simulink model "test_increase_button_general"  (R2022b)
settings: Solver=FixedStepAuto  StartTime=0.0  StopTime=240  FixedStep=0.1  RelTol=1e-3
settings Model: Creator=alewi  LastModifiedBy=cristian
settings ConfigComp: CovEnable=on  RecordCoverage=on  CovModelRefEnable=on

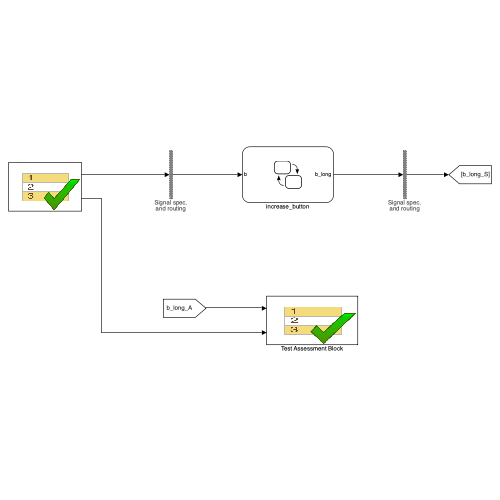
[thumbnail: Simulink's stored preview of the top-level diagram]
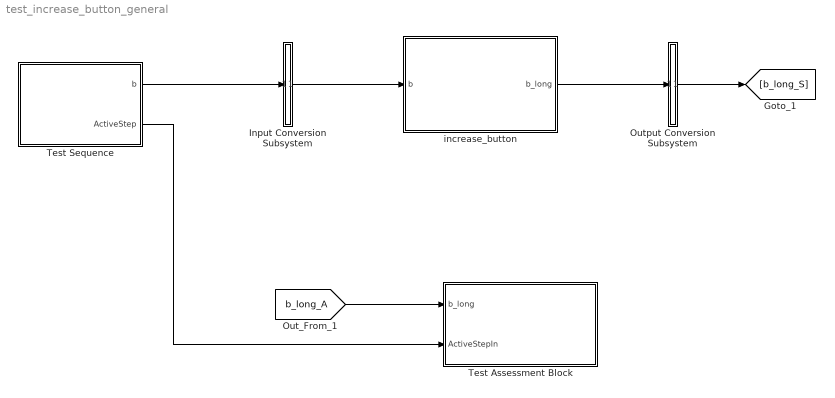
== system test_increase_button_general ==
  Input Conversion Subsystem : Subsystem  Tag=__SLT_ICS__  Description=|
      | Signal spec.
      | and routing
      settings: AttributesFormatString=%<Description>
  Output Conversion Subsystem : Subsystem  Tag=__SLT_OCS__  Description=|
      | Signal spec.
      | and routing
      settings: AttributesFormatString=%<Description>
  Test Assessment Block : Test Sequence  Tag=__SLT_ASMT__  TreatAsAtomicUnit=on
  Test Sequence : Test Sequence  TreatAsAtomicUnit=on
  increase_button : Stateflow chart  TreatAsAtomicUnit=on
  wires:
  Test Sequence/1(b) -> Input Conversion Subsystem/1(Inport_1)
  Output Conversion Subsystem/1(Outport_1) -> [b_long_S]
  Input Conversion Subsystem/1(Outport_1) -> increase_button/1(b)
  increase_button/1(b_long) -> Output Conversion Subsystem/1(Inport_1)
  Test Sequence/2(ActiveStep) -> Test Assessment Block/2(ActiveStepIn)
  [b_long_A] -> Test Assessment Block/1(b_long)

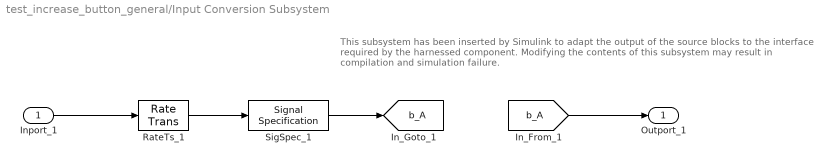
== system test_increase_button_general/Input Conversion Subsystem ==
  note: This subsystem has been inserted by Simulink to adapt the output of the source blocks to the interface required by the harnessed component.
      |  Modifying the contents of this subsystem may result in compilation and simulation failure.
  Inport_1 : Inport
  RateTs_1 : RateTransition  OutPortSampleTime=[-1, 0]
  SigSpec_1 : SignalSpecification  OutDataTypeStr=boolean  Dimensions=[1]  SampleTime=[-1, 0]
  Outport_1 : Outport
  tag scope: b_A=global
  wires:
  [b_A] -> Outport_1/1
  SigSpec_1/1 -> [b_A]
  RateTs_1/1 -> SigSpec_1/1
  Inport_1/1 -> RateTs_1/1

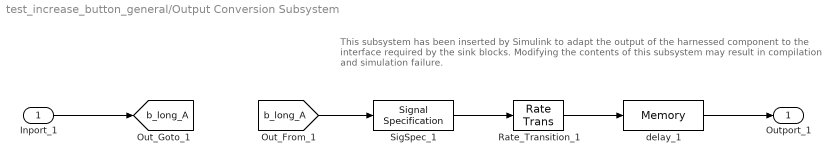
== system test_increase_button_general/Output Conversion Subsystem ==
  note: This subsystem has been inserted by Simulink to adapt the output of the harnessed component to the interface required by the sink blocks.
      |  Modifying the contents of this subsystem may result in compilation and simulation failure.
  Inport_1 : Inport
  Rate_Transition_1 : RateTransition  OutPortSampleTimeOpt=Inherit
  SigSpec_1 : SignalSpecification  OutDataTypeStr=boolean  Dimensions=[1]
  delay_1 : Memory
  Outport_1 : Outport
  tag scope: b_long_A=global
  wires:
  Inport_1/1 -> [b_long_A]
  [b_long_A] -> SigSpec_1/1
  SigSpec_1/1 -> Rate_Transition_1/1
  Rate_Transition_1/1 -> delay_1/1
  delay_1/1 -> Outport_1/1

== stateflow chart test_increase_button_general/Test Assessment Block ==
  state General
    state Run
      settings: description=Esecuzione test
      state Verify_G_Init
        verify(b_long == 1);
        settings: description=Inizialmente il bottone è rilasciato, per cui non è stato rilevato alcun long press.
      state Verify_G_ButtonPressed1
        settings: description=Bottone premuto
        state Verify_G_ButtonPressed1_1
          verify(b_long == 1);
          settings: description=Fino a che non passa 1 secondo, non viene rilevato alcun cambiamento nella potenza.
        state Verify_G_ButtonPressed1_2
          verify(b_long == 0);
          settings: description=Viene rilevata la pressione lunga.
        (default) -> Verify_G_ButtonPressed1_1
        Verify_G_ButtonPressed1_1 -> Verify_G_ButtonPressed1_2 : [
            | after(1,sec)
            | ]
      state Verify_G_ButtonReleased
        verify(b_long == 1);
        settings: description=La pressione lunga viene resettata.
      state Verify_G_ButtonPressed2
        settings: description=Bottone premuto
        state Verify_G_ButtonPressed2_1
          verify(b_long == 1)
          settings: description=Fino a che non passa 1 secondo, non viene rilevato alcun cambiamento nella potenza.
        state Verify_G_ButtonPressed2_2
          verify(b_long == 0);
          settings: description=Viene rilevata la pressione lunga.
        state Verify_G_ButtonPressed2_3
          verify(b_long == 1)
          settings: description=La pressione lunga viene resettata.
        (default) -> Verify_G_ButtonPressed2_1
        Verify_G_ButtonPressed2_1 -> Verify_G_ButtonPressed2_2 : [
            | after(1,sec)
            | ]
        Verify_G_ButtonPressed2_2 -> Verify_G_ButtonPressed2_3 : [
            | after(sampleTime,sec)
            | ]
      state Verify_G_ButtonReleased2
        verify(b_long == 1)
        settings: description=Il bottone è rilasciato, per cui non viene rilevato alcun long press
      state step_1_2
      (default) -> (junction 311)
      Run -> (junction 311)
      (junction 311) -> (junction 312) [order 1] : [ActiveStepIn == ActiveStepEnumH1.G_Init
          | ]
      (junction 312) -> Verify_G_Init [order 1] : [~in(General.Run.Verify_G_Init)]
      (junction 311) -> (junction 320) [order 2]
      (junction 312) -> (junction 315) [order 2]
      (junction 320) -> (junction 321) [order 1] : [ActiveStepIn == ActiveStepEnumH1.G_ButtonPressed
          | ]
      (junction 321) -> Verify_G_ButtonPressed1 [order 1] : [~in(General.Run.Verify_G_ButtonPressed1)]
      (junction 320) -> (junction 335) [order 2]
      (junction 321) -> (junction 324) [order 2]
      (junction 335) -> (junction 336) [order 1] : [ActiveStepIn == ActiveStepEnumH1.G_ButtonReleased
          | ]
      (junction 336) -> Verify_G_ButtonReleased [order 1] : [~in(General.Run.Verify_G_ButtonReleased)]
      (junction 335) -> (junction 343) [order 2]
      (junction 336) -> (junction 339) [order 2]
      (junction 343) -> (junction 344) [order 1] : [ActiveStepIn == ActiveStepEnumH1.G_ButtonPressed2
          | ]
      (junction 344) -> Verify_G_ButtonPressed2 [order 1] : [~in(General.Run.Verify_G_ButtonPressed2)]
      (junction 343) -> (junction 384) [order 2]
      (junction 344) -> (junction 347) [order 2]
      (junction 384) -> (junction 385) [order 1] : [ActiveStepIn == ActiveStepEnumH1.G_ButtonReleased2
          | ]
      (junction 385) -> Verify_G_ButtonReleased2 [order 1] : [~in(General.Run.Verify_G_ButtonReleased2)]
      (junction 384) -> (junction 351) [order 2]
      (junction 385) -> (junction 388) [order 2]
      (junction 351) -> (junction 352)
      (junction 352) -> step_1_2 [order 1] : [~in(General.Run.step_1_2)]
      (junction 352) -> (junction 355) [order 2]
    (default) -> Run
  (default) -> General : {assert(Active_Scenario_Index == 1,'The value of Scenario Parameter ''Active_Scenario_Index'' is not valid. Use the index of the scenario to specify it.')}
  data: b_long input boolean size=[1]; ActiveStepIn input; Active_Scenario_Index parameter =1; sampleTime constant double =str2num(get_param('InductionCooker','FixedStep'))

== stateflow chart test_increase_button_general/Test Sequence ==
  settings: updateMethod=DISCRETE  sampleTime=0.1
  state General
    state G_Init
      %% Initialize data outputs.
      b = true;
      settings: description=|
          | Pulsante non premuto.
          | Il pulsante lavora in logica negata come avviene per il bottone presente sulla scheda.
    state G_ButtonPressed
      b = false
      settings: description=|
          | Pulsante premuto.
          | Consideriamo questo step attivo per 1 secondo.
          | Attiva la transizione da Wait a Pressed.
    state G_ButtonReleased
      b = true
      settings: description=|
          | Pulsante rilasciato.
          | Ci aspettiamo che sia stata rilevata la richiesta di aumento della potenza.
          | Il pulsante torna nello stato di Wait, attivando la transizione da Pressed a Wait.
    state G_ButtonPressed2
      b = false
      settings: description=|
          | Pulsante premuto a lungo.
          | Prima passa da Wait a Pressed e poi da Pressed a LongPressed.
    state G_ButtonReleased2
      b = true
      settings: description=|
          | Pulsante rilasciato.
          | Passa da LongPressed a Wait.
    (default) -> G_Init
    G_Init -> G_ButtonPressed : [
        | true
        | ]
    G_ButtonPressed -> G_ButtonReleased : [
        | after(1+ sampleTime,sec)
        | ]
    G_ButtonReleased -> G_ButtonPressed2 : [
        | after(0.1,sec)
        | ]
    G_ButtonPressed2 -> G_ButtonReleased2 : [
        | after(2+ sampleTime,sec)
        | ]
  (default) -> General : {assert(Active_Scenario_Index == 1,'The value of Scenario Parameter ''Active_Scenario_Index'' is not valid. Use the index of the scenario to specify it.')}
  data: b output boolean size=[1]; ActiveStep output Enum: ActiveStepEnumH1; sampleTime constant double =str2num(get_param('InductionCooker','FixedStep')); Active_Scenario_Index parameter =1

== stateflow chart test_increase_button_general/increase_button ==
  note: Bottone a livelli, la pressione per un numero di secondi pari a DURATION permette di avere un uscita alta in maniera istantanea.
      | Per avere in output un valore PRESSED, è necessare lasciare il bottone e premere tra un output e l'altro.
  state Wait
    en: b_long = RELEASED
  state Pressed
    en: b_long = RELEASED;
    on after(DURATION,sec): b_long = PRESSED
  state LongPressed
    en: b_long = RELEASED
  (default) -> Wait
  Wait -> Pressed : [b == PRESSED]
  Pressed -> Wait [order 1] : [b == RELEASED]
  LongPressed -> Wait : [b == RELEASED]
  Pressed -> LongPressed [order 2] : [b_long == PRESSED && b == PRESSED]
  data: b_long output boolean size=1; PRESSED constant boolean size=1 =0; RELEASED constant boolean size=1 =1; b input boolean size=1; DURATION constant double size=1 =1
